simulink model "schSimuSegway_2018a"  (R2018b)
settings: Solver=VariableStepAuto  StartTime=0.0  StopTime=tfinal  RelTol=1e-3
InitFcn:
  | disp('init inports and outports numbers');
  | in_cb=1;
  | in_cm=2;
  | in_um=3;
  | out_thb=1;
  | out_thm=2;
  | out_vb=3;
  | out_vm=4;
  | out_um=5;
  | if exist('G')~=1
  | %--------------------------------------------------
  | % valeurs des parametres par defaut
  | %--------------------------------------------------
  | disp('init default parameters');
  | time_values_cb=[0,0];
  | time_values_cm=[0,0];
  | time_values_um=[0,0];
  | tfinal=10;
  | thm_init=0*pi/180;vthm_init=0*pi/180;
  | thb_init=0*pi/180;vthb_init=0*pi/180;
  | %------------------------------------------------------------------
  | % parametres des moteurs FIT0450U d'entrainement du segway en deplacement rectiligne
  | % dans ce cas les 2 moteurs sont attaques par la meme tension d'induit Um
  | %-----------------------------------------------------------------
  | 
  | Im=2*0.0061; % inertie de 2 moteurs en sortie de reducteur, ne devrait pas etre negligable !...
  | Kem= 0.277; % rapport fcem / vitesse en sortie de reducteur :V/(rd/s)=Nm/A;
  | 
  | Kim=2 *0.277;% 2. rapport couple  en sortie de reducteur/ courant :Nm/A = V/(rd/s);
  | Rm=2.8;% resistance d'induit en ohm
  | fm=2* 0.0108;% frottement visqueux en sortie de reducteur
  | u_max=5; % tension max des moteurs
  | u_dead=0.5; % bande morte due au frottement sec en volt
  | %------------------------------------------------------------------
  | % parametres mecanique du segway
  | %-----------------------------------------------------------------
  | G=9.81; % acceleration gravite terrestre en m/s2
  | % barre
  | Mb= 0.277; %Masse segway sans batterie 277g
  | Lb =  0.056000; % distance essieu centre de masse en m
  | Ib=1e-4 ; % inertie de la barre autour de son centre de masse en Kg.m^2
  | % batterie
  | Mbat=2*0.096; %masse en Kg des 2  batteries VoltCraft 5000 de 96g chacune
  | LxBat=0.022;LyBat=2*0.036;LzBat=0.075;
  | Ibat=1/12*Mbat*(LyBat^2+LzBat^2); % inertie batt/ centre de masse batt en kg.m2
  | Lbat=0.085;%0.085; % distance essieu centre de masse Batteries
  | %roues
  | Rr=0.07; % rayon des roues en m
  | Mr=2 * 0; % masse de 2 roues, negligable
  | Ir=1/2*Rr^2*Mr; % inertie des 2 roues, =1 cylindre plein de masse Mr, de rayon Rr autour de son axe de rotation
  | I1=Ir+(Mb+Mr+Mbat)*Rr^2; %avec Batterie
  | Ieb=Ib+Ibat+Mb*Lb^2+Mbat*Lbat^2;% avec Batterie
  | 
  | 
  | end
values from neighbouring files (symbols this model uses):
  K = [-22.0083946552 -0.385164851676 -3.66015572739 -0.971821179518]    [Kplace.mat]    (also in convertToParallelCells.m = 0; paralellCells.m = 0; programme_segway_etudiant.m = place(A,BUm,poles_BF))
  Kem = 0.277    [programme_segway_etudiant.m]
settings Model: Creator=sygorra  LastModifiedBy=maitrise
settings DataIOCC: SaveFormat=Array

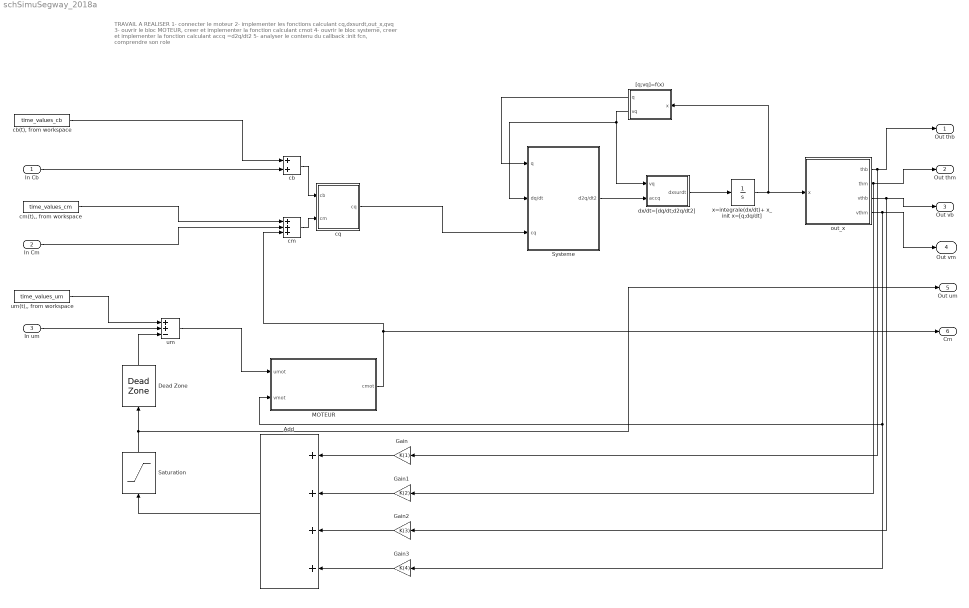
== system schSimuSegway_2018a ==
  note: TRAVAIL A REALISER
      | 1- connecter le moteur
      | 2- implementer les fonctions calculant cq,dxsurdt,out_x,qvq
      | 3- ouvrir le bloc MOTEUR, creer et implementer la fonction calculant cmot
      | 4- ouvrir le bloc systeme, creer et implementer la fonction calculant accq =d2q/dt2
      | 5- analyser le contenu du callback :init fcn, comprendre son role
  In Cb : Inport
  In Cm : Inport  Port=2
  In um : Inport  Port=3
  Add : Sum  Inputs=++++
  Dead Zone : DeadZone  LowerValue=-u_dead  UpperValue=u_dead  SaturateOnIntegerOverflow=on
  Gain : Gain  Gain=K(1)
  Gain1 : Gain  Gain=K(2)
  Gain2 : Gain  Gain=K(3)
  Gain3 : Gain  Gain=K(4)
  MOTEUR : Subsystem
  Saturation : Saturate  UpperLimit=u_max  LowerLimit=-u_max
  Systeme : Subsystem
  "[q;vq]=f(x)" : MATLAB Function  TreatAsAtomicUnit=on
  cb : Sum
  "cb(t), from workspace" : FromWorkspace  VariableName=time_values_cb  SampleTime=0
  cm : Sum  Inputs=+++
  "cm(t),, from workspace" : FromWorkspace  VariableName=time_values_cm  SampleTime=0
  cq : MATLAB Function  TreatAsAtomicUnit=on
  dx/dt=[dq/dt;d2q/dt2] : MATLAB Function  TreatAsAtomicUnit=on
  out_x : MATLAB Function  TreatAsAtomicUnit=on
  "um " : Sum  Inputs=++-
  "um(t),, from workspace" : FromWorkspace  VariableName=time_values_um  SampleTime=0
  x=integrale(dx/dt)+ x_init x=[q;dq/dt] : Integrator  InitialCondition=[thb_init;thm_init;vthb_init;vthm_init]
  Out thb : Outport
  Out thm : Outport  Port=2
  Out vb : Outport  Port=3
  Out vm : Outport  Port=4
  Out um : Outport  Port=5
  "Cm " : Outport  Port=6
  wires:
  "cb(t), from workspace"/1 -> cb/1
  In Cb/1 -> cb/2
  In um/1 -> "um "/2
  "um(t),, from workspace"/1 -> "um "/1
  In Cm/1 -> cm/2
  "cm(t),, from workspace"/1 -> cm/1
  cb/1 -> cq/1(cb)
  cm/1 -> cq/2(cm)
  cq/1(cq) -> Systeme/3(cq)
  x=integrale(dx/dt)+ x_init x=[q;dq/dt]/1 -> "[q;vq]=f(x)"/1(x), out_x/1(x)
  "[q;vq]=f(x)"/1(q) -> Systeme/1(q)
  "[q;vq]=f(x)"/2(vq) -> dx/dt=[dq/dt;d2q/dt2]/1(vq), Systeme/2(dq/dt)
  dx/dt=[dq/dt;d2q/dt2]/1(dxsurdt) -> x=integrale(dx/dt)+ x_init x=[q;dq/dt]/1
  Systeme/1(d2q/dt2) -> dx/dt=[dq/dt;d2q/dt2]/2(accq)
  out_x/1(thb) -> Gain/1, Out thb/1
  out_x/2(thm) -> Gain1/1, Out thm/1
  out_x/3(vthb) -> Gain2/1, Out vb/1
  out_x/4(vthm) -> Gain3/1, MOTEUR/2(vmot), Out vm/1
  "um "/1 -> MOTEUR/1(umot)
  MOTEUR/1(cmot) -> "Cm "/1, cm/3
  Gain/1 -> Add/1
  Gain1/1 -> Add/2
  Gain2/1 -> Add/3
  Gain3/1 -> Add/4
  Add/1 -> Saturation/1
  Dead Zone/1 -> "um "/3
  Saturation/1 -> Out um/1, Dead Zone/1

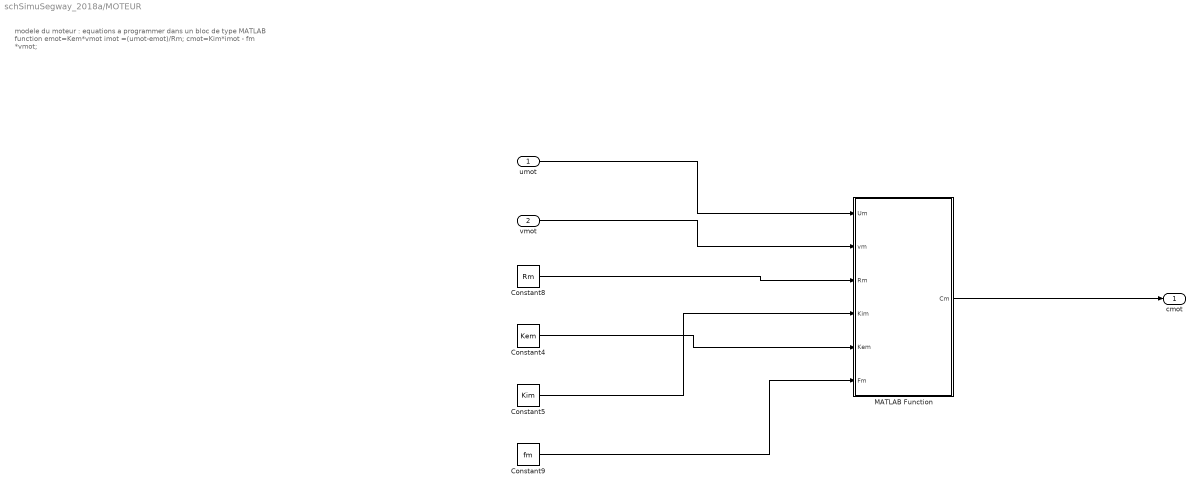
== system schSimuSegway_2018a/MOTEUR ==
  note: modele du moteur : equations a programmer dans un bloc de type MATLAB function
      | emot=Kem*vmot
      | imot =(umot-emot)/Rm;
      | cmot=Kim*imot - fm *vmot;
  umot : Inport
  vmot : Inport  Port=2
  Constant4 : Constant  Value=Kem
  Constant5 : Constant  Value=Kim
  Constant8 : Constant  Value=Rm
  Constant9 : Constant  Value=fm
  MATLAB Function : MATLAB Function  TreatAsAtomicUnit=on
  cmot : Outport  VectorParamsAs1DForOutWhenUnconnected=on
  wires:
  umot/1 -> MATLAB Function/1(Um)
  Constant5/1 -> MATLAB Function/4(Kim)
  Constant8/1 -> MATLAB Function/3(Rm)
  vmot/1 -> MATLAB Function/2(vm)
  Constant4/1 -> MATLAB Function/5(Kem)
  Constant9/1 -> MATLAB Function/6(Fm)
  MATLAB Function/1(Cm) -> cmot/1

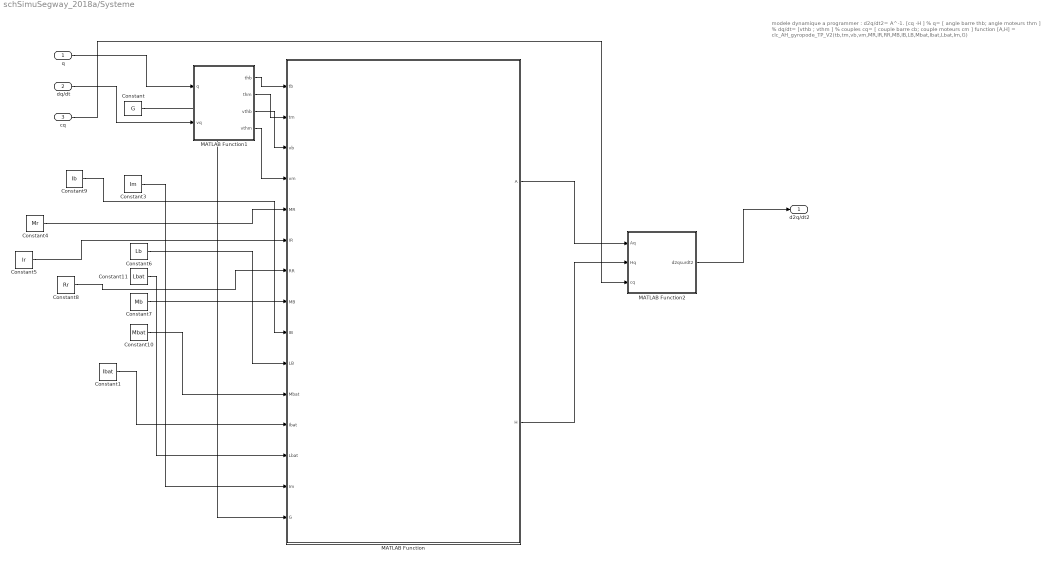
== system schSimuSegway_2018a/Systeme ==
  note: modele dynamique a programmer : d2q/dt2= A^-1. [cq -H ]
      |
      | % q= [ angle barre thb; angle moteurs thm ]
      | % dq/dt= [vthb ; vthm ]
      | % couples cq= [ couple barre cb; couple moteurs cm ]
      | function [A,H] = clc_AH_gyropode_TP_V2(tb,tm,vb,vm,MR,IR,RR,MB,IB,LB,Mbat,Ibat,Lbat,Im,G)
  q : Inport
  dq/dt : Inport  Port=2
  cq : Inport  Port=3
  Constant : Constant  Value=G
  Constant1 : Constant  Value=Ibat
  Constant10 : Constant  Value=Mbat
  Constant11 : Constant  Value=Lbat
  Constant3 : Constant  Value=Im
  Constant4 : Constant  Value=Mr
  Constant5 : Constant  Value=Ir
  Constant6 : Constant  Value=Lb
  Constant7 : Constant  Value=Mb
  Constant8 : Constant  Value=Rr
  Constant9 : Constant  Value=Ib
  MATLAB Function : MATLAB Function  TreatAsAtomicUnit=on
  MATLAB Function1 : MATLAB Function  TreatAsAtomicUnit=on
  MATLAB Function2 : MATLAB Function  TreatAsAtomicUnit=on
  d2q/dt2 : Outport
  wires:
  Constant/1 -> MATLAB Function/15(G)
  Constant6/1 -> MATLAB Function/10(LB)
  Constant7/1 -> MATLAB Function/8(MB)
  Constant10/1 -> MATLAB Function/11(Mbat)
  Constant3/1 -> MATLAB Function/14(Im)
  Constant11/1 -> MATLAB Function/13(Lbat)
  MATLAB Function/2(H) -> MATLAB Function2/2(Hq)
  MATLAB Function/1(A) -> MATLAB Function2/1(Aq)
  cq/1 -> MATLAB Function2/3(cq)
  MATLAB Function2/1(d2qsurdt2) -> d2q/dt2/1
  q/1 -> MATLAB Function1/1(q)
  dq/dt/1 -> MATLAB Function1/2(vq)
  MATLAB Function1/2(thm) -> MATLAB Function/2(tm)
  MATLAB Function1/1(thb) -> MATLAB Function/1(tb)
  MATLAB Function1/4(vthm) -> MATLAB Function/4(vm)
  MATLAB Function1/3(vthb) -> MATLAB Function/3(vb)
  Constant4/1 -> MATLAB Function/5(MR)
  Constant5/1 -> MATLAB Function/6(IR)
  Constant8/1 -> MATLAB Function/7(RR)
  Constant9/1 -> MATLAB Function/9(IB)
  Constant1/1 -> MATLAB Function/12(Ibat)

== matlab function schSimuSegway_2018a/cq ==
  data: cb input; cm input; cq output
function cq=fcn(cb,cm)

cq= [cb;cm];

== matlab function schSimuSegway_2018a/Systeme/MATLAB Function ==
  data: tb input; A output; tm input; vb input; vm input; MR input; IR input; RR input; MB input; IB input; LB input; Mbat input; Ibat input; Lbat input; Im input; G input; H output
function [A,H] = clc_AH(tb,tm,vb,vm,MR,IR,RR,MB,IB,LB,Mbat,Ibat,Lbat,Im,G)
 [A,H] = clc_AH_gyropode_TP_V2(tb,tm,vb,vm,MR,IR,RR,MB,IB,LB,Mbat,Ibat,Lbat,Im,G);

== matlab function schSimuSegway_2018a/[q;vq]=f(x) ==
  data: x input; q output; vq output
function [q,vq] =qvq_(x)

q=x(1:2,1);
vq=x(3:4,1);

== matlab function schSimuSegway_2018a/dx//dt=[dq//dt;d2q//dt2] ==
  data: vq input; dxsurdt output; accq input
function dxsurdt  =vx_(vq,accq)

dxsurdt=[vq;accq];

== matlab function schSimuSegway_2018a/out_x ==
  data: x input; thb output; thm output; vthb output; vthm output
function [thb,thm,vthb,vthm] =outputs_(x)

thb=x(1,1);
thm=x(2,1);
vthb=x(3,1); 
vthm=x(4,1);

== matlab function schSimuSegway_2018a/Systeme/MATLAB Function1 ==
  data: thb output; q input; vq input; thm output; vthb output; vthm output
function [thb,thm,vthb,vthm]= fcn(q,vq)

thb = q(1,1); 
thm = q(2,1);  
vthb = vq(1,1); 
vthm = vq(2,1);

== matlab function schSimuSegway_2018a/Systeme/MATLAB Function2 ==
  data: Aq input; d2qsurdt2 output; Hq input; cq input
function d2qsurdt2 = d2qsurdt2_(Aq,Hq,cq)

%d2qsurdt2 = inv(Aq)*(cq-Hq); 
d2qsurdt2 = Aq\(cq - Hq); % il est preferable d'ecrire ça dans ce cas

== matlab function schSimuSegway_2018a/MOTEUR/MATLAB Function ==
  data: Um input; Cm output; vm input; Rm input; Kim input; Kem input; Fm input
function Cm  = fcn(Um,vm,Rm,Kim,Kem,Fm) 

Em = Kem*vm; 
Im = (Um - Em)/Rm ; 
Cm= Kim*Im - Fm*vm ;
